simulink model "plant"  (Simulink 7.9)
settings: Solver=ode45  StartTime=0.0  StopTime=40  RelTol=1e-3
values from neighbouring files (symbols this model uses):
  A = [1 2 0; 3 1 -2; 4 -2 1]    [calcul_gains.m]    (also in script.m; script1.m)
  B = [1; -1; 1]    [calcul_gains.m]    (also in script.m; script1.m)
  Bd = [0; 1; 0]    [calcul_gains.m]    (also in script.m; script1.m)
  C = [7 8 1]    [calcul_gains.m]    (also in script.m; script1.m)
  D = 0    [calcul_gains.m]    (also in script.m; script1.m)
  dbar = 0    [script.m]    (also in script1.m)
  Dd = 0    [calcul_gains.m]    (also in script.m; script1.m)
  ubar = xubar(4)    [script.m]    (also in script1.m)
  xbar = xubar(1:3)    [script.m]    (also in script1.m)
libraries: simulink x1
settings Model: Creator=PhM  LastModifiedBy=PhM
settings OptimizationCC: InitFltsAndDblsToZero=on
settings DebuggingCC: SaveWithParameterizedLinksMsg=none  SignalResolutionControl=TryResolveAllWithWarning  MultiTaskDSMMsg=warning  MultiTaskCondExecSysMsg=none  FcnCallInpInsideContextMsg=Use local settings  StrictBusMsg=None
settings RTWCC: IncludeERTFirstTime=on
settings GRTTargetCC: TargetFcnLib=ansi_tfl_tmw.mat  CombineOutputUpdateFcns=off  GRTInterface=on

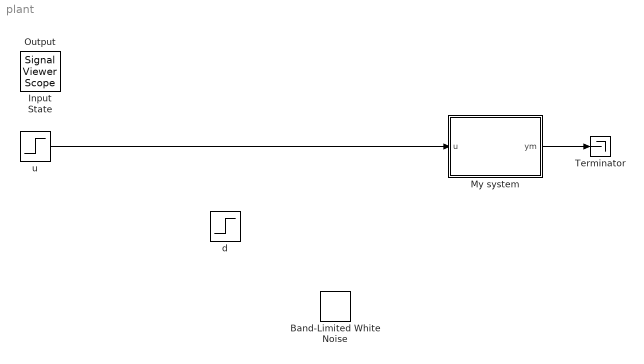
== system plant ==
  My system : Subsystem
  Terminator : Terminator
  u : Step  Time=5  Before=ubar  After=ubar+1  SampleTime=0
  Band-Limited White Noise : simulink/Sources/Band-Limited White Noise  IOType=siggen  Cov=1e-6  Ts=1e-3  seed=[23341]
  Input : SignalViewerScope  IOType=viewer  NumInputPorts=2  LegendLocations="0.72634     0.90311     0.19753    0.035179 0.72788     0.44204     0.19753    0.035179"  RefreshTime=0.035000
      settings: ShowLegends=on  TimeRange=40  YMin=0.2~0  YMax=1.6~0.05  SaveName=ScopeData2
  Output : SignalViewerScope  IOType=viewer  NumInputPorts=2  RefreshTime=0.035000
      settings: TimeRange=10  YMin=-3e+006~-3e+006  YMax=500000~500000
  State : SignalViewerScope  IOType=viewer  ZoomMode=yonly  RefreshTime=0.035000
      settings: TimeRange=10  YMin=-300000  YMax=200000
  d : Step  IOType=siggen  Time=10  Before=dbar  After=dbar+0.05  SampleTime=0
  wires:
  u/1 -> My system/1(u)
  My system/1(ym) -> Terminator/1

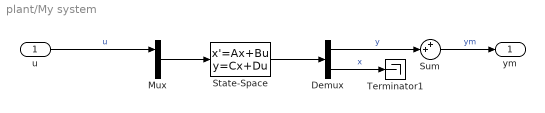
== system plant/My system ==
  u : Inport
  Demux : Demux  Outputs=[1 3]
  Mux : Mux  Inputs=2
  State-Space : StateSpace  A=A  B=[B Bd]  C=[C; eye(3)]  D=[D Dd; zeros(3,2)]  X0=xbar
  Sum : Sum  Inputs=++|
  Terminator1 : Terminator
  ym : Outport
  wires:
  Mux/1 -> State-Space/1
  State-Space/1 -> Demux/1
  Demux/1 -> Sum/2  "y"
  Demux/2 -> Terminator1/1  "x"
  u/1 -> Mux/1  "u"
  Sum/1 -> ym/1  "ym"
